simulink model "psbsyncmachine"  (Simulink 6.0)
settings: Solver=ode15s  SolverMode=SingleTasking  StartTime=0.0  StopTime=3  FixedStep=300e-6  RelTol=1e-3
InitFcn:
  | powericon('psbinitsys',bdroot);
libraries: powerlib2 x9, powerlib_extras x1
settings Model: Creator=patrice  LastModifiedBy=batserve  ExtModeTrigMode=oneshot  ExtModeArmWhenConnect=off  ExtModeAutoUpdateStatusClock=off
settings DataIOCC: InitialState=xFinal  LimitDataPoints=off  SaveOutput=off  TimeSaveName=t  SignalLoggingName=sigsOut
settings OptimizationCC: BlockReduction=off  BooleanDataType=off
settings DebuggingCC: SolverPrmCheckMsg=none  UnconnectedInputMsg=none  UnconnectedOutputMsg=none
settings HardwareCC: TargetUnknown=on
settings RTWCC: TemplateMakefile=grt_unix.tmf

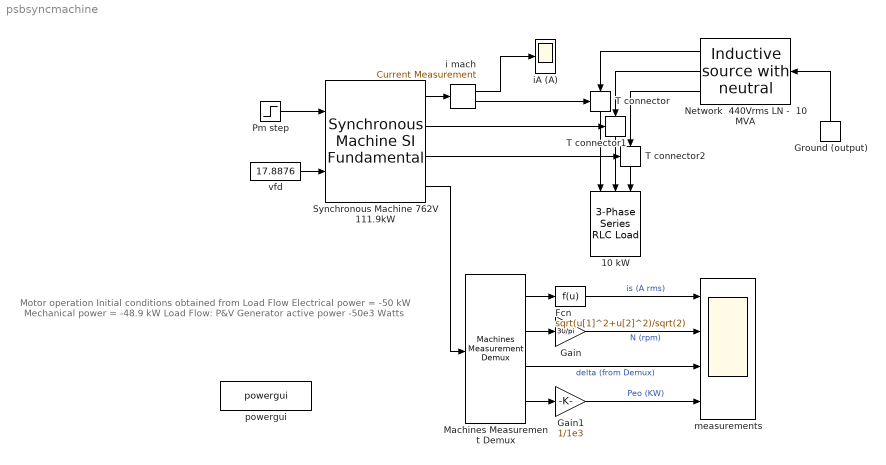
== system psbsyncmachine ==
  note: Motor operation
      | Initial  conditions obtained from Load Flow
      | Electrical power =  -50 kW
      | Mechanical power = -48.9 kW
      |
      | Load Flow:
      | P&V Generator
      | active power -50e3 Watts
  10 kW : powerlib2/Elements/3-Phase Series RLC Load  Orientation=down  Vpp=762  fn=60  P3=10e3  QL3=0  QC3=0
  Fcn : Fcn  Expr=sqrt(u[1]^2+u[2]^2)/sqrt(2)
  Gain : Gain  Gain=30/pi  SaturateOnIntegerOverflow=on
  Gain1 : Gain  Gain=1/1e3  SaturateOnIntegerOverflow=on
  Ground (output) : powerlib2/Connectors/Ground (output)  Tag=PoWeRsYsTeMbLoCk  Orientation=up  PSBOutputType=1
  Machines Measurement Demux : powerlib2/Machines/Machines Measurement Demux  machType=Synchronous  ssm1=on  ssm2=on  ssm3=on  ssm4=on  ssm5=on  ssm6=on  sm1=off  sm2=on  sm3=off  sm4=off  sm5=off  sm6=off  sm7=off  sm8=on  sm9=off  sm10=off  sm11=off  sm115=off  sm12=on  sm13=on  sm14=off  asm1=on  asm2=on  asm3=on  asm4=on  asm5=on  asm6=on  asm7=on  asm8=on  asm9=on  asm10=on  asm11=on  pmsm1=on  pmsm2=on  pmsm3=on  pmsm4=on  pmsm5=on  pmsm6=on  lastType=1
  Network  440Vrms LN -  10 MVA : powerlib_extras/Three-Phase Library/Inductive source with neutral  Orientation=left  V=440*sqrt(2)  Phi=0  F=60  R=762^2/10e6/10  L=762^2/10e6/(2*pi*60)
  Pm step : Step  Time=0.1  Before=-48863  After=-60000  SampleTime=0
  Synchronous Machine 762V 111.9kW : powerlib2/Machines/Synchronous Machine SI Fundamental  Tag=PoWeRsYsTeMbLoCk  rotorType=Salient-pole  x1="[ 111.9e3 440*sqrt(3)  60  0]"  x2=[ .26 1.14e-3 13.7e-3 11.0e-3 ]  x3=[ 0.13 2.1e-3 ]  x4b=[ 1 2 3 4 5 6 ]  x4=[ 0.0224 1.4e-3 0.02 1e-3 ]  x5=[ 24.9 0 2 ]  x6=[0 -111.483 53.9768 53.9768 53.9768 -173.297 66.7033 -53.2967 17.8876]  x7=off  x8=[]  x9=off  PSBOutputType=1110  iounits=1  LoadFlowParameters=[1,0,0,0,0]
  T connector : powerlib2/Connectors/T connector  Tag=PoWeRsYsTeMbLoCk  Orientation=down  PSBOutputType=1
  T connector1 : powerlib2/Connectors/T connector  Tag=PoWeRsYsTeMbLoCk  Orientation=down  PSBOutputType=1
  T connector2 : powerlib2/Connectors/T connector  Tag=PoWeRsYsTeMbLoCk  Orientation=down  PSBOutputType=1
  i mach : powerlib2/Measurements/Current Measurement  Tag=PoWeRsYsTeMmEaSuReMeNt  PhasorSimulation=off  OutputType=Magnitude  PSBOutputType=01  PSBequivalent=0
  iA (A) : Scope
      settings: TickLabels=on  TimeRange=1  YMin=430  YMax=520  SaveName=is1  DataFormat=Array
  measurements : Scope  NumInputPorts=4
      settings: TickLabels=on  TimeRange=1  YMin=38~-5~-5~-5  YMax=53~5~5~5  SaveName=is2
  powergui : powerlib2/powergui  Frange=logspace(0,3,50)  Ylog=off  Xlog=off  save=off  variable=ZData  ZoomFFT=on  StartTime=0.0  cycles=2  DisplayStyle=off  fundamental=60  FreqAxis=off  MaxFrequency=1000  frequencyindice=1  frequencyindicesteady=1  RmsSteady=1  display=off  Ts=0  methode=off  frequency=60  echomessages=off
  vfd : Constant  Value=17.8876
  wires:
  Synchronous Machine 762V 111.9kW/4 -> Machines Measurement Demux/1
  vfd/1 -> Synchronous Machine 762V 111.9kW/2
  Synchronous Machine 762V 111.9kW/1 -> i mach/1
  Pm step/1 -> Synchronous Machine 762V 111.9kW/1
  Fcn/1 -> measurements/1  "is (A rms)"
  Machines Measurement Demux/1 -> Fcn/1
  Machines Measurement Demux/2 -> Gain/1
  Gain/1 -> measurements/2  "N (rpm)"
  Ground (output)/1 -> Network  440Vrms LN -  10 MVA/1
  i mach/2 -> T connector/Enable
  Network  440Vrms LN -  10 MVA/1 -> T connector/1
  T connector/1 -> 10 kW/1
  Synchronous Machine 762V 111.9kW/2 -> T connector1/Enable
  Network  440Vrms LN -  10 MVA/2 -> T connector1/1
  T connector1/1 -> 10 kW/2
  Synchronous Machine 762V 111.9kW/3 -> T connector2/Enable
  T connector2/1 -> 10 kW/3
  Network  440Vrms LN -  10 MVA/3 -> T connector2/1
  i mach/1 -> iA (A)/1
  Machines Measurement Demux/3 -> measurements/3  "delta (from Demux)"
  Gain1/1 -> measurements/4  "Peo (KW)"
  Machines Measurement Demux/4 -> Gain1/1
